simulink model "vegas13_fastnettest_250mhz_r1"  (Simulink 7.4)
settings: Solver=ode45  StartTime=0.0  StopTime=20000  RelTol=1e-3
undefined symbols (not defined in the file or in its folder): ROACH
libraries: xbsIndex_r4 x179, xps_library x20, casper_library_misc x18, dspsigops x16, casper_library_flow_control x4
(part 2 of 3)

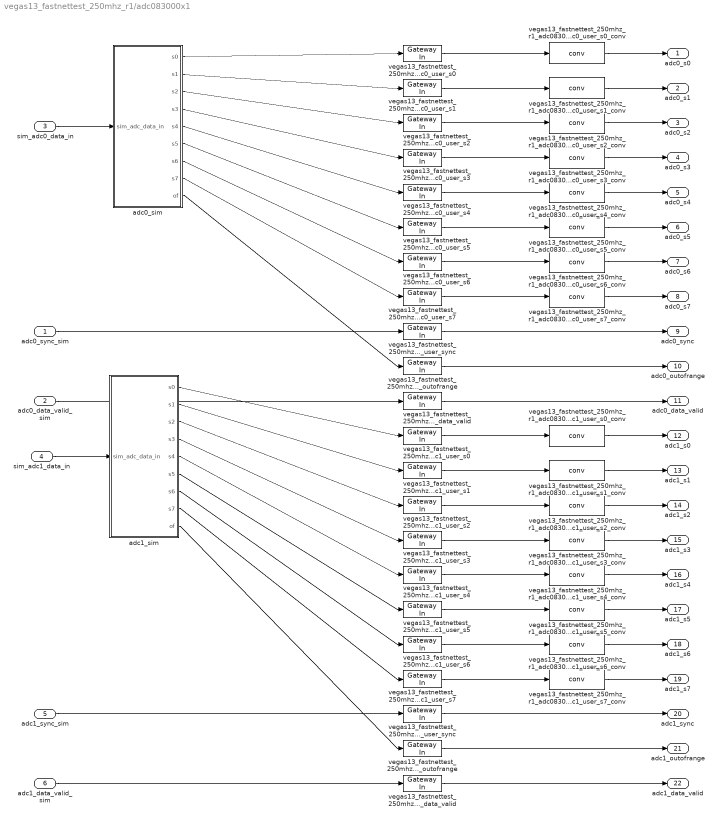
== system vegas13_fastnettest_250mhz_r1/adc083000x1 ==
  adc0_sync_sim : Inport  OutDataType=sfix(16)  OutScaling=2^0
  adc0_data_valid_sim : Inport  Port=2  OutDataType=sfix(16)  OutScaling=2^0
  sim_adc0_data_in : Inport  Port=3  OutDataType=fixdt(1, 16)  OutScaling=2^0
  sim_adc1_data_in : Inport  Port=4  OutDataType=fixdt(1, 16)  OutScaling=2^0
  adc1_sync_sim : Inport  Port=5  OutDataType=fixdt(1, 16)  OutScaling=2^0
  adc1_data_valid_sim : Inport  Port=6  OutDataType=fixdt(1, 16)  OutScaling=2^0
  adc0_sim : Subsystem  AncestorBlock=xps_library/ADCs/adc_sim  mask(adc_sim){nStreams=8, bit_width=8}
      mask prompts: nStreams "Number of Output Streams"; bit_width "Sample Bit Width"
      mask help:
      | This block simulates the behavior of a demuxed ADC, which takes
      | as input a waveform and returns digital samples in parallel at
      | a slower rate.
      |
      | This block is used to simulate the behavior
      mask init:
      | adc_sim_init(gcb, ...
      |     'nStreams', nStreams, ...
      |     'bit_width', bit_width);
  adc1_sim : Subsystem  AncestorBlock=xps_library/ADCs/adc_sim  mask(adc_sim){nStreams=8, bit_width=8}
      mask prompts: nStreams "Number of Output Streams"; bit_width "Sample Bit Width"
      mask help:
      | This block simulates the behavior of a demuxed ADC, which takes
      | as input a waveform and returns digital samples in parallel at
      | a slower rate.
      |
      | This block is used to simulate the behavior
      mask init:
      | adc_sim_init(gcb, ...
      |     'nStreams', nStreams, ...
      |     'bit_width', bit_width);
  vegas13_fastnettest_250mhz_r1_adc083000x1_adc0_user_data_valid : xbsIndex_r4/Gateway In  arith_type=Unsigned  n_bits=1  bin_pt=0  quantization="Round  (unbiased: +/- Inf)"  overflow=Saturate  period=1  dbl_ovrd=off  timing_constraint=None  locs_specified=off  LOCs={}  hdl_port=on  block_type=gatewayin
      settings: infoedit="Gateway in block.  Converts inputs of type Simulink integer, double and fixed point to  Xilinx fixed point type.<br><br>Hardware notes:  In hardware these blocks become top level input ports."  block_version=11.4
  vegas13_fastnettest_250mhz_r1_adc083000x1_adc0_user_outofrange : xbsIndex_r4/Gateway In  arith_type=Unsigned  n_bits=4  bin_pt=0  quantization="Round  (unbiased: +/- Inf)"  overflow=Saturate  period=1  dbl_ovrd=off  timing_constraint=None  locs_specified=off  LOCs={}  hdl_port=on  block_type=gatewayin
      settings: infoedit="Gateway in block.  Converts inputs of type Simulink integer, double and fixed point to  Xilinx fixed point type.<br><br>Hardware notes:  In hardware these blocks become top level input ports."  block_version=11.4
  vegas13_fastnettest_250mhz_r1_adc083000x1_adc0_user_s{0..7} (8 alike) : xbsIndex_r4/Gateway In  arith_type=Unsigned  n_bits=8  bin_pt=0  quantization="Round  (unbiased: +/- Inf)"  overflow=Saturate  period=1  dbl_ovrd=off  timing_constraint=None  locs_specified=off  LOCs={}  hdl_port=on  block_type=gatewayin
      settings: infoedit="Gateway in block.  Converts inputs of type Simulink integer, double and fixed point to  Xilinx fixed point type.<br><br>Hardware notes:  In hardware these blocks become top level input ports."  block_version=11.4
  vegas13_fastnettest_250mhz_r1_adc083000x1_adc0_user_s0_conv : xps_library/ADCs/conv  SystemSampleTime=-1  bit_width=8
  vegas13_fastnettest_250mhz_r1_adc083000x1_adc0_user_s1_conv : xps_library/ADCs/conv  SystemSampleTime=-1  bit_width=8
  vegas13_fastnettest_250mhz_r1_adc083000x1_adc0_user_s2_conv : xps_library/ADCs/conv  SystemSampleTime=-1  bit_width=8
  vegas13_fastnettest_250mhz_r1_adc083000x1_adc0_user_s3_conv : xps_library/ADCs/conv  SystemSampleTime=-1  bit_width=8
  vegas13_fastnettest_250mhz_r1_adc083000x1_adc0_user_s4_conv : xps_library/ADCs/conv  SystemSampleTime=-1  bit_width=8
  vegas13_fastnettest_250mhz_r1_adc083000x1_adc0_user_s5_conv : xps_library/ADCs/conv  SystemSampleTime=-1  bit_width=8
  vegas13_fastnettest_250mhz_r1_adc083000x1_adc0_user_s6_conv : xps_library/ADCs/conv  SystemSampleTime=-1  bit_width=8
  vegas13_fastnettest_250mhz_r1_adc083000x1_adc0_user_s7_conv : xps_library/ADCs/conv  SystemSampleTime=-1  bit_width=8
  vegas13_fastnettest_250mhz_r1_adc083000x1_adc0_user_sync : xbsIndex_r4/Gateway In  arith_type=Unsigned  n_bits=4  bin_pt=0  quantization="Round  (unbiased: +/- Inf)"  overflow=Saturate  period=1  dbl_ovrd=off  timing_constraint=None  locs_specified=off  LOCs={}  hdl_port=on  block_type=gatewayin
      settings: infoedit="Gateway in block.  Converts inputs of type Simulink integer, double and fixed point to  Xilinx fixed point type.<br><br>Hardware notes:  In hardware these blocks become top level input ports."  block_version=11.4
  vegas13_fastnettest_250mhz_r1_adc083000x1_adc1_user_data_valid : xbsIndex_r4/Gateway In  arith_type=Unsigned  n_bits=1  bin_pt=0  quantization="Round  (unbiased: +/- Inf)"  overflow=Saturate  period=1  dbl_ovrd=off  timing_constraint=None  locs_specified=off  LOCs={}  hdl_port=on  block_type=gatewayin
      settings: infoedit="Gateway in block.  Converts inputs of type Simulink integer, double and fixed point to  Xilinx fixed point type.<br><br>Hardware notes:  In hardware these blocks become top level input ports."  block_version=11.4
  vegas13_fastnettest_250mhz_r1_adc083000x1_adc1_user_outofrange : xbsIndex_r4/Gateway In  arith_type=Unsigned  n_bits=4  bin_pt=0  quantization="Round  (unbiased: +/- Inf)"  overflow=Saturate  period=1  dbl_ovrd=off  timing_constraint=None  locs_specified=off  LOCs={}  hdl_port=on  block_type=gatewayin
      settings: infoedit="Gateway in block.  Converts inputs of type Simulink integer, double and fixed point to  Xilinx fixed point type.<br><br>Hardware notes:  In hardware these blocks become top level input ports."  block_version=11.4
  vegas13_fastnettest_250mhz_r1_adc083000x1_adc1_user_s{0..7} (8 alike) : xbsIndex_r4/Gateway In  arith_type=Unsigned  n_bits=8  bin_pt=0  quantization="Round  (unbiased: +/- Inf)"  overflow=Saturate  period=1  dbl_ovrd=off  timing_constraint=None  locs_specified=off  LOCs={}  hdl_port=on  block_type=gatewayin
      settings: infoedit="Gateway in block.  Converts inputs of type Simulink integer, double and fixed point to  Xilinx fixed point type.<br><br>Hardware notes:  In hardware these blocks become top level input ports."  block_version=11.4
  vegas13_fastnettest_250mhz_r1_adc083000x1_adc1_user_s0_conv : xps_library/ADCs/conv  SystemSampleTime=-1  bit_width=8
  vegas13_fastnettest_250mhz_r1_adc083000x1_adc1_user_s1_conv : xps_library/ADCs/conv  SystemSampleTime=-1  bit_width=8
  vegas13_fastnettest_250mhz_r1_adc083000x1_adc1_user_s2_conv : xps_library/ADCs/conv  SystemSampleTime=-1  bit_width=8
  vegas13_fastnettest_250mhz_r1_adc083000x1_adc1_user_s3_conv : xps_library/ADCs/conv  SystemSampleTime=-1  bit_width=8
  vegas13_fastnettest_250mhz_r1_adc083000x1_adc1_user_s4_conv : xps_library/ADCs/conv  SystemSampleTime=-1  bit_width=8
  vegas13_fastnettest_250mhz_r1_adc083000x1_adc1_user_s5_conv : xps_library/ADCs/conv  SystemSampleTime=-1  bit_width=8
  vegas13_fastnettest_250mhz_r1_adc083000x1_adc1_user_s6_conv : xps_library/ADCs/conv  SystemSampleTime=-1  bit_width=8
  vegas13_fastnettest_250mhz_r1_adc083000x1_adc1_user_s7_conv : xps_library/ADCs/conv  SystemSampleTime=-1  bit_width=8
  vegas13_fastnettest_250mhz_r1_adc083000x1_adc1_user_sync : xbsIndex_r4/Gateway In  arith_type=Unsigned  n_bits=4  bin_pt=0  quantization="Round  (unbiased: +/- Inf)"  overflow=Saturate  period=1  dbl_ovrd=off  timing_constraint=None  locs_specified=off  LOCs={}  hdl_port=on  block_type=gatewayin
      settings: infoedit="Gateway in block.  Converts inputs of type Simulink integer, double and fixed point to  Xilinx fixed point type.<br><br>Hardware notes:  In hardware these blocks become top level input ports."  block_version=11.4
  adc0_s0 : Outport  OutDataType=fixdt(1, 16)  OutScaling=2^0
  adc0_s1 : Outport  Port=2  OutDataType=fixdt(1, 16)  OutScaling=2^0
  adc0_s2 : Outport  Port=3  OutDataType=fixdt(1, 16)  OutScaling=2^0
  adc0_s3 : Outport  Port=4  OutDataType=fixdt(1, 16)  OutScaling=2^0
  adc0_s4 : Outport  Port=5  OutDataType=fixdt(1, 16)  OutScaling=2^0
  adc0_s5 : Outport  Port=6  OutDataType=fixdt(1, 16)  OutScaling=2^0
  adc0_s6 : Outport  Port=7  OutDataType=fixdt(1, 16)  OutScaling=2^0
  adc0_s7 : Outport  Port=8  OutDataType=fixdt(1, 16)  OutScaling=2^0
  adc0_sync : Outport  Port=9  OutDataType=sfix(16)  OutScaling=2^0
  adc0_outofrange : Outport  Port=10  OutDataType=fixdt(1, 16)  OutScaling=2^0
  adc0_data_valid : Outport  Port=11  OutDataType=sfix(16)  OutScaling=2^0
  adc1_s0 : Outport  Port=12  OutDataType=fixdt(1, 16)  OutScaling=2^0
  adc1_s1 : Outport  Port=13  OutDataType=fixdt(1, 16)  OutScaling=2^0
  adc1_s2 : Outport  Port=14  OutDataType=fixdt(1, 16)  OutScaling=2^0
  adc1_s3 : Outport  Port=15  OutDataType=fixdt(1, 16)  OutScaling=2^0
  adc1_s4 : Outport  Port=16  OutDataType=fixdt(1, 16)  OutScaling=2^0
  adc1_s5 : Outport  Port=17  OutDataType=fixdt(1, 16)  OutScaling=2^0
  adc1_s6 : Outport  Port=18  OutDataType=fixdt(1, 16)  OutScaling=2^0
  adc1_s7 : Outport  Port=19  OutDataType=fixdt(1, 16)  OutScaling=2^0
  adc1_sync : Outport  Port=20  OutDataType=fixdt(1, 16)  OutScaling=2^0
  adc1_outofrange : Outport  Port=21  OutDataType=fixdt(1, 16)  OutScaling=2^0
  adc1_data_valid : Outport  Port=22  OutDataType=fixdt(1, 16)  OutScaling=2^0
  wires:
  sim_adc0_data_in/1 -> adc0_sim/1(sim_adc_data_in)
  sim_adc1_data_in/1 -> adc1_sim/1(sim_adc_data_in)
  adc0_sim/1(s0) -> vegas13_fastnettest_250mhz_r1_adc083000x1_adc0_user_s0/1
  vegas13_fastnettest_250mhz_r1_adc083000x1_adc0_user_s0/1 -> vegas13_fastnettest_250mhz_r1_adc083000x1_adc0_user_s0_conv/1
  vegas13_fastnettest_250mhz_r1_adc083000x1_adc0_user_s0_conv/1 -> adc0_s0/1
  adc0_sim/2(s1) -> vegas13_fastnettest_250mhz_r1_adc083000x1_adc0_user_s1/1
  vegas13_fastnettest_250mhz_r1_adc083000x1_adc0_user_s1/1 -> vegas13_fastnettest_250mhz_r1_adc083000x1_adc0_user_s1_conv/1
  vegas13_fastnettest_250mhz_r1_adc083000x1_adc0_user_s1_conv/1 -> adc0_s1/1
  adc0_sim/3(s2) -> vegas13_fastnettest_250mhz_r1_adc083000x1_adc0_user_s2/1
  vegas13_fastnettest_250mhz_r1_adc083000x1_adc0_user_s2/1 -> vegas13_fastnettest_250mhz_r1_adc083000x1_adc0_user_s2_conv/1
  vegas13_fastnettest_250mhz_r1_adc083000x1_adc0_user_s2_conv/1 -> adc0_s2/1
  adc0_sim/4(s3) -> vegas13_fastnettest_250mhz_r1_adc083000x1_adc0_user_s3/1
  vegas13_fastnettest_250mhz_r1_adc083000x1_adc0_user_s3/1 -> vegas13_fastnettest_250mhz_r1_adc083000x1_adc0_user_s3_conv/1
  vegas13_fastnettest_250mhz_r1_adc083000x1_adc0_user_s3_conv/1 -> adc0_s3/1
  adc0_sim/5(s4) -> vegas13_fastnettest_250mhz_r1_adc083000x1_adc0_user_s4/1
  vegas13_fastnettest_250mhz_r1_adc083000x1_adc0_user_s4/1 -> vegas13_fastnettest_250mhz_r1_adc083000x1_adc0_user_s4_conv/1
  vegas13_fastnettest_250mhz_r1_adc083000x1_adc0_user_s4_conv/1 -> adc0_s4/1
  adc0_sim/6(s5) -> vegas13_fastnettest_250mhz_r1_adc083000x1_adc0_user_s5/1
  vegas13_fastnettest_250mhz_r1_adc083000x1_adc0_user_s5/1 -> vegas13_fastnettest_250mhz_r1_adc083000x1_adc0_user_s5_conv/1
  vegas13_fastnettest_250mhz_r1_adc083000x1_adc0_user_s5_conv/1 -> adc0_s5/1
  adc0_sim/7(s6) -> vegas13_fastnettest_250mhz_r1_adc083000x1_adc0_user_s6/1
  vegas13_fastnettest_250mhz_r1_adc083000x1_adc0_user_s6/1 -> vegas13_fastnettest_250mhz_r1_adc083000x1_adc0_user_s6_conv/1
  vegas13_fastnettest_250mhz_r1_adc083000x1_adc0_user_s6_conv/1 -> adc0_s6/1
  adc0_sim/8(s7) -> vegas13_fastnettest_250mhz_r1_adc083000x1_adc0_user_s7/1
  vegas13_fastnettest_250mhz_r1_adc083000x1_adc0_user_s7/1 -> vegas13_fastnettest_250mhz_r1_adc083000x1_adc0_user_s7_conv/1
  vegas13_fastnettest_250mhz_r1_adc083000x1_adc0_user_s7_conv/1 -> adc0_s7/1
  adc0_sync_sim/1 -> vegas13_fastnettest_250mhz_r1_adc083000x1_adc0_user_sync/1
  vegas13_fastnettest_250mhz_r1_adc083000x1_adc0_user_sync/1 -> adc0_sync/1
  adc0_sim/9(of) -> vegas13_fastnettest_250mhz_r1_adc083000x1_adc0_user_outofrange/1
  vegas13_fastnettest_250mhz_r1_adc083000x1_adc0_user_outofrange/1 -> adc0_outofrange/1
  adc0_data_valid_sim/1 -> vegas13_fastnettest_250mhz_r1_adc083000x1_adc0_user_data_valid/1
  vegas13_fastnettest_250mhz_r1_adc083000x1_adc0_user_data_valid/1 -> adc0_data_valid/1
  adc1_sim/1(s0) -> vegas13_fastnettest_250mhz_r1_adc083000x1_adc1_user_s0/1
  vegas13_fastnettest_250mhz_r1_adc083000x1_adc1_user_s0/1 -> vegas13_fastnettest_250mhz_r1_adc083000x1_adc1_user_s0_conv/1
  vegas13_fastnettest_250mhz_r1_adc083000x1_adc1_user_s0_conv/1 -> adc1_s0/1
  adc1_sim/2(s1) -> vegas13_fastnettest_250mhz_r1_adc083000x1_adc1_user_s1/1
  vegas13_fastnettest_250mhz_r1_adc083000x1_adc1_user_s1/1 -> vegas13_fastnettest_250mhz_r1_adc083000x1_adc1_user_s1_conv/1
  vegas13_fastnettest_250mhz_r1_adc083000x1_adc1_user_s1_conv/1 -> adc1_s1/1
  adc1_sim/3(s2) -> vegas13_fastnettest_250mhz_r1_adc083000x1_adc1_user_s2/1
  vegas13_fastnettest_250mhz_r1_adc083000x1_adc1_user_s2/1 -> vegas13_fastnettest_250mhz_r1_adc083000x1_adc1_user_s2_conv/1
  vegas13_fastnettest_250mhz_r1_adc083000x1_adc1_user_s2_conv/1 -> adc1_s2/1
  adc1_sim/4(s3) -> vegas13_fastnettest_250mhz_r1_adc083000x1_adc1_user_s3/1
  vegas13_fastnettest_250mhz_r1_adc083000x1_adc1_user_s3/1 -> vegas13_fastnettest_250mhz_r1_adc083000x1_adc1_user_s3_conv/1
  vegas13_fastnettest_250mhz_r1_adc083000x1_adc1_user_s3_conv/1 -> adc1_s3/1
  adc1_sim/5(s4) -> vegas13_fastnettest_250mhz_r1_adc083000x1_adc1_user_s4/1
  vegas13_fastnettest_250mhz_r1_adc083000x1_adc1_user_s4/1 -> vegas13_fastnettest_250mhz_r1_adc083000x1_adc1_user_s4_conv/1
  vegas13_fastnettest_250mhz_r1_adc083000x1_adc1_user_s4_conv/1 -> adc1_s4/1
  adc1_sim/6(s5) -> vegas13_fastnettest_250mhz_r1_adc083000x1_adc1_user_s5/1
  vegas13_fastnettest_250mhz_r1_adc083000x1_adc1_user_s5/1 -> vegas13_fastnettest_250mhz_r1_adc083000x1_adc1_user_s5_conv/1
  vegas13_fastnettest_250mhz_r1_adc083000x1_adc1_user_s5_conv/1 -> adc1_s5/1
  adc1_sim/7(s6) -> vegas13_fastnettest_250mhz_r1_adc083000x1_adc1_user_s6/1
  vegas13_fastnettest_250mhz_r1_adc083000x1_adc1_user_s6/1 -> vegas13_fastnettest_250mhz_r1_adc083000x1_adc1_user_s6_conv/1
  vegas13_fastnettest_250mhz_r1_adc083000x1_adc1_user_s6_conv/1 -> adc1_s6/1
  adc1_sim/8(s7) -> vegas13_fastnettest_250mhz_r1_adc083000x1_adc1_user_s7/1
  vegas13_fastnettest_250mhz_r1_adc083000x1_adc1_user_s7/1 -> vegas13_fastnettest_250mhz_r1_adc083000x1_adc1_user_s7_conv/1
  vegas13_fastnettest_250mhz_r1_adc083000x1_adc1_user_s7_conv/1 -> adc1_s7/1
  adc1_sync_sim/1 -> vegas13_fastnettest_250mhz_r1_adc083000x1_adc1_user_sync/1
  vegas13_fastnettest_250mhz_r1_adc083000x1_adc1_user_sync/1 -> adc1_sync/1
  adc1_sim/9(of) -> vegas13_fastnettest_250mhz_r1_adc083000x1_adc1_user_outofrange/1
  vegas13_fastnettest_250mhz_r1_adc083000x1_adc1_user_outofrange/1 -> adc1_outofrange/1
  adc1_data_valid_sim/1 -> vegas13_fastnettest_250mhz_r1_adc083000x1_adc1_user_data_valid/1
  vegas13_fastnettest_250mhz_r1_adc083000x1_adc1_user_data_valid/1 -> adc1_data_valid/1

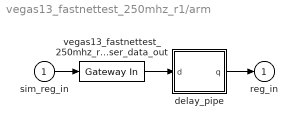
== system vegas13_fastnettest_250mhz_r1/arm ==
  sim_reg_in : Inport
  delay_pipe : Subsystem
  vegas13_fastnettest_250mhz_r1_arm_user_data_out : xbsIndex_r4/Gateway In  arith_type=Unsigned  n_bits=32  bin_pt=0  quantization="Round  (unbiased: +/- Inf)"  overflow=Saturate  period=1  dbl_ovrd=off  timing_constraint=None  locs_specified=off  LOCs={}  hdl_port=on  block_type=gatewayin
      settings: infoedit="Gateway in block.  Converts inputs of type Simulink integer, double and fixed point to  Xilinx fixed point type.<br><br>Hardware notes:  In hardware these blocks become top level input ports."  block_version=11.4
  reg_in : Outport
  wires:
  delay_pipe/1(q) -> reg_in/1
  vegas13_fastnettest_250mhz_r1_arm_user_data_out/1 -> delay_pipe/1(d)
  sim_reg_in/1 -> vegas13_fastnettest_250mhz_r1_arm_user_data_out/1

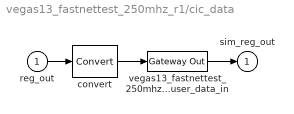
== system vegas13_fastnettest_250mhz_r1/cic_data ==
  reg_out : Inport
  convert : xbsIndex_r4/Convert  arith_type=Unsigned  n_bits=32  bin_pt=0  quantization=Truncate  overflow=Wrap  latency=0  dbl_ovrd=off  pipeline=off  block_type=convert
      settings: block_version=11.4
  vegas13_fastnettest_250mhz_r1_cic_data_user_data_in : xbsIndex_r4/Gateway Out  hdl_port=on  timing_constraint=None  locs_specified=off  LOCs={}  block_type=gatewayout
      settings: infoedit="Gateway out block.  Converts Xilinx fixed point inputs into ouputs of type Simulink integer, double, or fixed point.<br><br>Hardware notes:  In hardware these blocks become top level output ports or are discarded, depending on how they are configured."  block_version=11.4
  sim_reg_out : Outport
  wires:
  vegas13_fastnettest_250mhz_r1_cic_data_user_data_in/1 -> sim_reg_out/1
  convert/1 -> vegas13_fastnettest_250mhz_r1_cic_data_user_data_in/1
  reg_out/1 -> convert/1

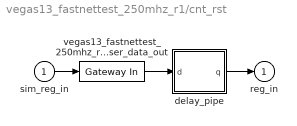
== system vegas13_fastnettest_250mhz_r1/cnt_rst ==
  sim_reg_in : Inport
  delay_pipe : Subsystem
  vegas13_fastnettest_250mhz_r1_cnt_rst_user_data_out : xbsIndex_r4/Gateway In  arith_type=Unsigned  n_bits=32  bin_pt=0  quantization="Round  (unbiased: +/- Inf)"  overflow=Saturate  period=1  dbl_ovrd=off  timing_constraint=None  locs_specified=off  LOCs={}  hdl_port=on  block_type=gatewayin
      settings: infoedit="Gateway in block.  Converts inputs of type Simulink integer, double and fixed point to  Xilinx fixed point type.<br><br>Hardware notes:  In hardware these blocks become top level input ports."  block_version=11.4
  reg_in : Outport
  wires:
  delay_pipe/1(q) -> reg_in/1
  vegas13_fastnettest_250mhz_r1_cnt_rst_user_data_out/1 -> delay_pipe/1(d)
  sim_reg_in/1 -> vegas13_fastnettest_250mhz_r1_cnt_rst_user_data_out/1

== system vegas13_fastnettest_250mhz_r1/dest_ip ==
  sim_reg_in : Inport
  delay_pipe : Subsystem
  vegas13_fastnettest_250mhz_r1_dest_ip_user_data_out : xbsIndex_r4/Gateway In  arith_type=Unsigned  n_bits=32  bin_pt=0  quantization="Round  (unbiased: +/- Inf)"  overflow=Saturate  period=1  dbl_ovrd=off  timing_constraint=None  locs_specified=off  LOCs={}  hdl_port=on  block_type=gatewayin
      settings: infoedit="Gateway in block.  Converts inputs of type Simulink integer, double and fixed point to  Xilinx fixed point type.<br><br>Hardware notes:  In hardware these blocks become top level input ports."  block_version=11.4
  reg_in : Outport
  wires:
  delay_pipe/1(q) -> reg_in/1
  vegas13_fastnettest_250mhz_r1_dest_ip_user_data_out/1 -> delay_pipe/1(d)
  sim_reg_in/1 -> vegas13_fastnettest_250mhz_r1_dest_ip_user_data_out/1

== system vegas13_fastnettest_250mhz_r1/dest_port ==
  sim_reg_in : Inport
  delay_pipe : Subsystem
  vegas13_fastnettest_250mhz_r1_dest_port_user_data_out : xbsIndex_r4/Gateway In  arith_type=Unsigned  n_bits=32  bin_pt=0  quantization="Round  (unbiased: +/- Inf)"  overflow=Saturate  period=1  dbl_ovrd=off  timing_constraint=None  locs_specified=off  LOCs={}  hdl_port=on  block_type=gatewayin
      settings: infoedit="Gateway in block.  Converts inputs of type Simulink integer, double and fixed point to  Xilinx fixed point type.<br><br>Hardware notes:  In hardware these blocks become top level input ports."  block_version=11.4
  reg_in : Outport
  wires:
  delay_pipe/1(q) -> reg_in/1
  vegas13_fastnettest_250mhz_r1_dest_port_user_data_out/1 -> delay_pipe/1(d)
  sim_reg_in/1 -> vegas13_fastnettest_250mhz_r1_dest_port_user_data_out/1

== system vegas13_fastnettest_250mhz_r1/eth_rst ==
  sim_reg_in : Inport
  delay_pipe : Subsystem
  vegas13_fastnettest_250mhz_r1_eth_rst_user_data_out : xbsIndex_r4/Gateway In  arith_type=Unsigned  n_bits=32  bin_pt=0  quantization="Round  (unbiased: +/- Inf)"  overflow=Saturate  period=1  dbl_ovrd=off  timing_constraint=None  locs_specified=off  LOCs={}  hdl_port=on  block_type=gatewayin
      settings: infoedit="Gateway in block.  Converts inputs of type Simulink integer, double and fixed point to  Xilinx fixed point type.<br><br>Hardware notes:  In hardware these blocks become top level input ports."  block_version=11.4
  reg_in : Outport
  wires:
  delay_pipe/1(q) -> reg_in/1
  vegas13_fastnettest_250mhz_r1_eth_rst_user_data_out/1 -> delay_pipe/1(d)
  sim_reg_in/1 -> vegas13_fastnettest_250mhz_r1_eth_rst_user_data_out/1

== system vegas13_fastnettest_250mhz_r1/ext_sync_ctr ==
  reg_out : Inport
  convert : xbsIndex_r4/Convert  arith_type=Unsigned  n_bits=32  bin_pt=0  quantization=Truncate  overflow=Wrap  latency=0  dbl_ovrd=off  pipeline=off  block_type=convert
      settings: block_version=11.4
  vegas13_fastnettest_250mhz_r1_ext_sync_ctr_user_data_in : xbsIndex_r4/Gateway Out  hdl_port=on  timing_constraint=None  locs_specified=off  LOCs={}  block_type=gatewayout
      settings: infoedit="Gateway out block.  Converts Xilinx fixed point inputs into ouputs of type Simulink integer, double, or fixed point.<br><br>Hardware notes:  In hardware these blocks become top level output ports or are discarded, depending on how they are configured."  block_version=11.4
  sim_reg_out : Outport
  wires:
  vegas13_fastnettest_250mhz_r1_ext_sync_ctr_user_data_in/1 -> sim_reg_out/1
  convert/1 -> vegas13_fastnettest_250mhz_r1_ext_sync_ctr_user_data_in/1
  reg_out/1 -> convert/1

== system vegas13_fastnettest_250mhz_r1/ip_select ==
  sim_reg_in : Inport
  delay_pipe : Subsystem
  vegas13_fastnettest_250mhz_r1_ip_select_user_data_out : xbsIndex_r4/Gateway In  arith_type=Unsigned  n_bits=32  bin_pt=0  quantization="Round  (unbiased: +/- Inf)"  overflow=Saturate  period=1  dbl_ovrd=off  timing_constraint=None  locs_specified=off  LOCs={}  hdl_port=on  block_type=gatewayin
      settings: infoedit="Gateway in block.  Converts inputs of type Simulink integer, double and fixed point to  Xilinx fixed point type.<br><br>Hardware notes:  In hardware these blocks become top level input ports."  block_version=11.4
  reg_in : Outport
  wires:
  delay_pipe/1(q) -> reg_in/1
  vegas13_fastnettest_250mhz_r1_ip_select_user_data_out/1 -> delay_pipe/1(d)
  sim_reg_in/1 -> vegas13_fastnettest_250mhz_r1_ip_select_user_data_out/1

== system vegas13_fastnettest_250mhz_r1/pkt_data ==
  reg_out : Inport
  convert : xbsIndex_r4/Convert  arith_type=Unsigned  n_bits=32  bin_pt=0  quantization=Truncate  overflow=Wrap  latency=0  dbl_ovrd=off  pipeline=off  block_type=convert
      settings: block_version=11.4
  vegas13_fastnettest_250mhz_r1_pkt_data_user_data_in : xbsIndex_r4/Gateway Out  hdl_port=on  timing_constraint=None  locs_specified=off  LOCs={}  block_type=gatewayout
      settings: infoedit="Gateway out block.  Converts Xilinx fixed point inputs into ouputs of type Simulink integer, double, or fixed point.<br><br>Hardware notes:  In hardware these blocks become top level output ports or are discarded, depending on how they are configured."  block_version=11.4
  sim_reg_out : Outport
  wires:
  vegas13_fastnettest_250mhz_r1_pkt_data_user_data_in/1 -> sim_reg_out/1
  convert/1 -> vegas13_fastnettest_250mhz_r1_pkt_data_user_data_in/1
  reg_out/1 -> convert/1

== system vegas13_fastnettest_250mhz_r1/port_select ==
  sim_reg_in : Inport
  delay_pipe : Subsystem
  vegas13_fastnettest_250mhz_r1_port_select_user_data_out : xbsIndex_r4/Gateway In  arith_type=Unsigned  n_bits=32  bin_pt=0  quantization="Round  (unbiased: +/- Inf)"  overflow=Saturate  period=1  dbl_ovrd=off  timing_constraint=None  locs_specified=off  LOCs={}  hdl_port=on  block_type=gatewayin
      settings: infoedit="Gateway in block.  Converts inputs of type Simulink integer, double and fixed point to  Xilinx fixed point type.<br><br>Hardware notes:  In hardware these blocks become top level input ports."  block_version=11.4
  reg_in : Outport
  wires:
  delay_pipe/1(q) -> reg_in/1
  vegas13_fastnettest_250mhz_r1_port_select_user_data_out/1 -> delay_pipe/1(d)
  sim_reg_in/1 -> vegas13_fastnettest_250mhz_r1_port_select_user_data_out/1

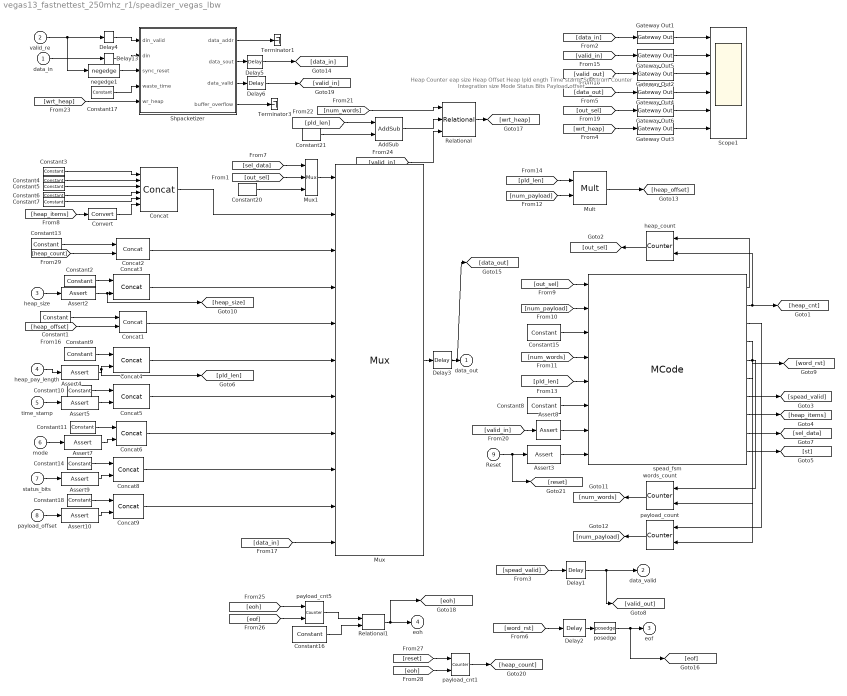
== system vegas13_fastnettest_250mhz_r1/speadizer_vegas_lbw ==
  note: Heap Counter
      | eap size
      | Heap Offset
      | Heap lpld ength
      | Time stamp
      | Spectrum Counter
      | Integration size
      | Mode
      | Status Bits
      | Payload offset
  data_in : Inport
  valid_re : Inport  Port=2
  heap_size : Inport  Port=3
  heap_pay_length : Inport  Port=4
  time_stamp : Inport  Port=5
  mode : Inport  Port=6
  status_bits : Inport  Port=7
  payload_offset : Inport  Port=8
  Reset : Inport  Port=9
  AddSub : xbsIndex_r4/AddSub  mode=Subtraction  use_carryin=off  use_carryout=off  en=off  latency=0  precision=Full  arith_type=Unsigned  n_bits=16  bin_pt=14  quantization=Truncate  overflow=Wrap  dbl_ovrd=off  use_behavioral_HDL=off  hw_selection=Fabric  pipelined=off  block_type=addsub
  Assert{2,4..5,7,9..10} (6 alike) : xbsIndex_r4/Assert  assert_type=on  type_source=Explicitly  arith_type=Unsigned  n_bits=spead_lsw  bin_pt=0  assert_rate=off  rate_source=Explicitly  period=1  output_port=on  block_type=assert
      settings: block_version=11.4
  Assert3 : xbsIndex_r4/Assert  assert_type=on  type_source=Explicitly  arith_type=Boolean  n_bits=spead_lsw  bin_pt=0  assert_rate=on  rate_source=Explicitly  period=1  output_port=on  block_type=assert
      settings: block_version=11.4
  Assert8 : xbsIndex_r4/Assert  assert_type=on  type_source=Explicitly  arith_type=Boolean  n_bits=spead_lsw  bin_pt=0  assert_rate=on  rate_source=Explicitly  period=1  output_port=on  block_type=assert
      settings: block_version=11.4
  Concat : xbsIndex_r4/Concat  num_inputs=6  dbl_ovrd=off  block_type=concat
  Concat{1..6,8..9} (8 alike) : xbsIndex_r4/Concat  num_inputs=2  dbl_ovrd=off  block_type=concat
  Constant1 : xbsIndex_r4/Constant  arith_type=Unsigned  const=8388608+3  n_bits=spead_msw  bin_pt=0  explicit_period=on  period=1  equ=P=C  opselect=C  inp2=PCIN>>17  opr=+  inp1=P  carry=CIN  dbl_ovrd=off  block_type=constant
      settings: block_version=11.4
  Constant10 : xbsIndex_r4/Constant  arith_type=Unsigned  const=8388608+32  n_bits=spead_msw  bin_pt=0  explicit_period=on  period=1  equ=P=C  opselect=C  inp2=PCIN>>17  opr=+  inp1=P  carry=CIN  dbl_ovrd=off  block_type=constant
      settings: block_version=11.4
  Constant11 : xbsIndex_r4/Constant  arith_type=Unsigned  const=8388608+33  n_bits=spead_msw  bin_pt=0  explicit_period=on  period=1  equ=P=C  opselect=C  inp2=PCIN>>17  opr=+  inp1=P  carry=CIN  dbl_ovrd=off  block_type=constant
      settings: block_version=11.4
  Constant13 : xbsIndex_r4/Constant  arith_type=Unsigned  const=8388608+1  n_bits=spead_msw  bin_pt=0  explicit_period=on  period=1  equ=P=C  opselect=C  inp2=PCIN>>17  opr=+  inp1=P  carry=CIN  dbl_ovrd=off  block_type=constant
      settings: block_version=11.4
  Constant14 : xbsIndex_r4/Constant  arith_type=Unsigned  const=8388608+34  n_bits=spead_msw  bin_pt=0  explicit_period=on  period=1  equ=P=C  opselect=C  inp2=PCIN>>17  opr=+  inp1=P  carry=CIN  dbl_ovrd=off  block_type=constant
      settings: block_version=11.4
  Constant15 : xbsIndex_r4/Constant  arith_type=Unsigned  const=num_items+5  n_bits=8  bin_pt=0  explicit_period=on  period=1  equ=P=C  opselect=C  inp2=PCIN>>17  opr=+  inp1=P  carry=CIN  dbl_ovrd=off  block_type=constant
      settings: block_version=11.4
  Constant16 : xbsIndex_r4/Constant  arith_type=Unsigned  const=num_payloads  n_bits=4  bin_pt=0  explicit_period=on  period=1  equ=P=C  opselect=C  inp2=PCIN>>17  opr=+  inp1=P  carry=CIN  dbl_ovrd=off  block_type=constant
      settings: block_version=11.4
  Constant17 : xbsIndex_r4/Constant  arith_type=Unsigned  const=pktzr_waste_time  n_bits=7  bin_pt=0  explicit_period=on  period=1  equ=P=C  opselect=C  inp2=PCIN>>17  opr=+  inp1=P  carry=CIN  dbl_ovrd=off  block_type=constant
  Constant18 : xbsIndex_r4/Constant  arith_type=Unsigned  const=0+35  n_bits=spead_msw  bin_pt=0  explicit_period=on  period=1  equ=P=C  opselect=C  inp2=PCIN>>17  opr=+  inp1=P  carry=CIN  dbl_ovrd=off  block_type=constant
      settings: block_version=11.4
  Constant2 : xbsIndex_r4/Constant  arith_type=Unsigned  const=8388608+2  n_bits=spead_msw  bin_pt=0  explicit_period=on  period=1  equ=P=C  opselect=C  inp2=PCIN>>17  opr=+  inp1=P  carry=CIN  dbl_ovrd=off  block_type=constant
      settings: block_version=11.4
  Constant20 : xbsIndex_r4/Constant  arith_type=Unsigned  const=num_items+5  n_bits=4  bin_pt=0  explicit_period=on  period=1  equ=P=C  opselect=C  inp2=PCIN>>17  opr=+  inp1=P  carry=CIN  dbl_ovrd=off  block_type=constant
      settings: block_version=11.4
  Constant21 : xbsIndex_r4/Constant  arith_type=Unsigned  const=16  n_bits=5  bin_pt=0  explicit_period=on  period=1  equ=P=C  opselect=C  inp2=PCIN>>17  opr=+  inp1=P  carry=CIN  dbl_ovrd=off  block_type=constant
      settings: block_version=11.4
  Constant3 : xbsIndex_r4/Constant  arith_type=Unsigned  const=83  n_bits=8  bin_pt=0  explicit_period=on  period=1  equ=P=C  opselect=C  inp2=PCIN>>17  opr=+  inp1=P  carry=CIN  dbl_ovrd=off  block_type=constant
      settings: block_version=11.4
  Constant4 : xbsIndex_r4/Constant  arith_type=Unsigned  const=4  n_bits=8  bin_pt=0  explicit_period=on  period=1  equ=P=C  opselect=C  inp2=PCIN>>17  opr=+  inp1=P  carry=CIN  dbl_ovrd=off  block_type=constant
      settings: block_version=11.4
  Constant5 : xbsIndex_r4/Constant  arith_type=Unsigned  const=3  n_bits=8  bin_pt=0  explicit_period=on  period=1  equ=P=C  opselect=C  inp2=PCIN>>17  opr=+  inp1=P  carry=CIN  dbl_ovrd=off  block_type=constant
      settings: block_version=11.4
  Constant6 : xbsIndex_r4/Constant  arith_type=Unsigned  const=5  n_bits=8  bin_pt=0  explicit_period=on  period=1  equ=P=C  opselect=C  inp2=PCIN>>17  opr=+  inp1=P  carry=CIN  dbl_ovrd=off  block_type=constant
      settings: block_version=11.4
  Constant7 : xbsIndex_r4/Constant  arith_type=Unsigned  const=0  n_bits=16  bin_pt=0  explicit_period=on  period=1  equ=P=C  opselect=C  inp2=PCIN>>17  opr=+  inp1=P  carry=CIN  dbl_ovrd=off  block_type=constant
      settings: block_version=11.4
  Constant8 : xbsIndex_r4/Constant  arith_type=Unsigned  const=num_payloads  n_bits=8  bin_pt=0  explicit_period=on  period=1  equ=P=C  opselect=C  inp2=PCIN>>17  opr=+  inp1=P  carry=CIN  dbl_ovrd=off  block_type=constant
      settings: block_version=11.4
  Constant9 : xbsIndex_r4/Constant  arith_type=Unsigned  const=8388608+4  n_bits=spead_msw  bin_pt=0  explicit_period=on  period=1  equ=P=C  opselect=C  inp2=PCIN>>17  opr=+  inp1=P  carry=CIN  dbl_ovrd=off  block_type=constant
      settings: block_version=11.4
  Convert : xbsIndex_r4/Convert  arith_type=Unsigned  n_bits=16  bin_pt=0  quantization=Truncate  overflow=Wrap  latency=0  dbl_ovrd=off  pipeline=off  block_type=convert
      settings: block_version=11.4
  Delay1 : xbsIndex_r4/Delay  en=off  latency=2  dbl_ovrd=off  reg_retiming=on  block_type=delay
      settings: block_version=11.4
  Delay13 : xbsIndex_r4/Delay  en=off  latency=2  dbl_ovrd=off  reg_retiming=off  block_type=delay
      settings: block_version=11.4
  Delay2 : xbsIndex_r4/Delay  en=off  latency=1  dbl_ovrd=off  reg_retiming=on  block_type=delay
      settings: block_version=11.4
  Delay3 : xbsIndex_r4/Delay  en=off  latency=1  dbl_ovrd=off  reg_retiming=on  block_type=delay
      settings: block_version=11.4
  Delay4 : xbsIndex_r4/Delay  en=off  latency=2  dbl_ovrd=off  reg_retiming=off  block_type=delay
      settings: block_version=11.4
  Delay5 : xbsIndex_r4/Delay  en=off  latency=3  dbl_ovrd=off  reg_retiming=on  block_type=delay
      settings: block_version=11.4
  Delay6 : xbsIndex_r4/Delay  en=off  latency=3  dbl_ovrd=off  reg_retiming=on  block_type=delay
      settings: block_version=11.4
  Gateway Out{1..6} (6 alike) : xbsIndex_r4/Gateway Out  hdl_port=on  timing_constraint=None  locs_specified=off  LOCs={}  block_type=gatewayout
      settings: infoedit="Gateway out block.  Converts Xilinx fixed point inputs into ouputs of type Simulink integer, double, or fixed point.<br><br>Hardware notes:  In hardware these blocks become top level output ports or are discarded, depending on how they are configured."  block_version=11.4
  Mult : xbsIndex_r4/Mult  precision=User Defined  arith_type=Unsigned  n_bits=40  bin_pt=0  quantization=Truncate  overflow=Wrap  en=off  latency=6  dbl_ovrd=off  use_behavioral_HDL=off  opt=Speed  use_embedded=on  optimum_pipeline=off  pipeline=on  use_rpm=on  placement_style=Triangular  block_type=mult
      settings: block_version=11.4
  Mux : xbsIndex_r4/Mux  inputs=10  en=off  latency=1  precision=User Defined  arith_type=Unsigned  n_bits=64  bin_pt=0  quantization=Truncate  overflow=Wrap  dbl_ovrd=off  block_type=mux
      settings: block_version=11.4
  Mux1 : xbsIndex_r4/Mux  inputs=2  en=off  latency=0  precision=Full  arith_type="Signed  (2's comp)"  n_bits=8  bin_pt=2  quantization=Truncate  overflow=Wrap  dbl_ovrd=off  block_type=mux
      settings: block_version=11.4
  Relational : xbsIndex_r4/Relational  mode=a>=b  en=on  latency=1  dbl_ovrd=off  block_type=relational
  Relational1 : xbsIndex_r4/Relational  mode=a=b  en=off  latency=0  dbl_ovrd=off  block_type=relational
  Scope1 : Scope  NumInputPorts=6
      settings: TimeRange=1000  YMin=0~0~0~0~0~0  YMax=40~1~1~1e+19~1~20  SaveName=ScopeData2  MaxDataPoints=10000
  Shpacketizer : Subsystem  AncestorBlock=gbt_library/Spacketizer  mask(shpacketizer){pin_width=256, sout_width=64, fifo_depth=128, total_words=1024}
      mask prompts: pin_width "Parallel Input Width"; sout_width "Serial Output Width"; fifo_depth "FIFO depth"; total_words "Total number of data points"
      mask help:
      | This block is intended to serialize data that is 'bursty', that is,
      | the average data rate is small but per cycle the data is highly
      | parallel and can contain many points simultaneously.  This situation
      | is common with the streaming CASPER FFTs and related blocks.
      |
      | The serialization buffers the data when valid and independently
      | serializes the data when the buffer is non-empty.  For convenience, the
      | data is counted as it is serialized and signals exist to indicate
      | that the serial output is valid or that a buffer overflow has occured.  The
      | block will not stop in the case of an overflow, and the overflow
      | signal is not held high after it occurs.
      |
      | For example usage, see 'roach_spec_2adc_borph' in 'SVNROOT/trunk/projects/roach_spec/'
      | or the test case in 'SVNROOT/trunk/mlib_devel_10_1/Tests/packetizer_test.mdl'
      |
      | For extended documentation, please see the CASPER wiki
      mask init:
      | shpacketizer_init(gcb, 'pin_width', pin_width, 'sout_width', sout_width, 'total_words', total_words, 'fifo_depth', fifo_depth)
      | % packetizer_init(gcb, ...
      | %     'pin_width', pin_width, ...
      | %     'sout_width', sout_width, ...
      | %   %  'fifo_depth', fifo_depth, ...
      | %     'total_words', total_words);
      settings: AttributesFormatString=|
      | Parallel Input Width: 256
      | Serial Output Width: 64
      mask StyleString: edit,edit,popup(16|32|64|128|256|512|1K|2K|4K|8K|16K|32K|64K),edit
  Terminator1 : Terminator
  Terminator3 : Terminator
  heap_count : xbsIndex_r4/Counter  cnt_type=Free Running  cnt_to=Inf  operation=Up  start_count=0  cnt_by_val=1  arith_type=Unsigned  n_bits=4  bin_pt=0  load_pin=off  rst=on  en=on  explicit_period=on  period=1  dbl_ovrd=off  use_behavioral_HDL=off  implementation=Fabric  block_type=counter
      settings: block_version=11.4
  negedge1 : casper_library_misc/negedge  Tag=Rising Edge Detector  SystemSampleTime=-1
  payload_cnt1 : xbsIndex_r4/Counter  cnt_type=Free Running  cnt_to=0  operation=Up  start_count=1024  cnt_by_val=1  arith_type=Unsigned  n_bits=40  bin_pt=0  load_pin=off  rst=on  en=on  explicit_period=on  period=1  dbl_ovrd=off  use_behavioral_HDL=off  implementation=Fabric  use_rpm=on  block_type=counter
      settings: xl_area=[0, 0, 0, 0, 0, 0, 0]
  payload_cnt5 : xbsIndex_r4/Counter  cnt_type=Free Running  cnt_to=0  operation=Up  start_count=0  cnt_by_val=1  arith_type=Unsigned  n_bits=4  bin_pt=0  load_pin=off  rst=on  en=on  explicit_period=on  period=1  dbl_ovrd=off  use_behavioral_HDL=off  implementation=Fabric  use_rpm=on  block_type=counter
      settings: xl_area=[0, 0, 0, 0, 0, 0, 0]
  payload_count : xbsIndex_r4/Counter  cnt_type=Free Running  cnt_to=Inf  operation=Up  start_count=0  cnt_by_val=1  arith_type=Unsigned  n_bits=8  bin_pt=0  load_pin=off  rst=on  en=on  explicit_period=on  period=1  dbl_ovrd=off  use_behavioral_HDL=off  implementation=Fabric  block_type=counter
      settings: block_version=11.4
  posedge : casper_library_misc/posedge  Tag=Rising Edge Detector  SystemSampleTime=-1
  spead_fsm : xbsIndex_r4/MCode  mfname=spead_fsm  explicit_period=on  period=1  inputsTable={'boundInpExpr'=>['','','','5','','','','',''],'inputs'=>['head_count','num_payload_sent','total_header_len','min_header_len','num_words_sent','payload_len','total_num_payloads','data_valid_in','rst']}  outputsTable={'outputs'=>['head_count_rst','head_count_en','num_payload_rst','num_payload_en','words_sent_rst','words_sent_en','tge_valid','heap_elements','select_data','st'],'suppressOut'=>['off','off','off','off','off','off','off','off','off','off']}  dbl_ovrd=off  enable_stdout=off  enable_debug=off  suppress_output=on  defparams={'min_header_len',5}  hide_port_list={}  block_type=mcode
      settings: block_version=11.4
  words_count : xbsIndex_r4/Counter  cnt_type=Free Running  cnt_to=Inf  operation=Up  start_count=0  cnt_by_val=8  arith_type=Unsigned  n_bits=15  bin_pt=0  load_pin=off  rst=on  en=on  explicit_period=on  period=1  dbl_ovrd=off  use_behavioral_HDL=off  implementation=Fabric  block_type=counter
      settings: block_version=11.4
  data_out : Outport
  data_valid : Outport  Port=2
  eof : Outport  Port=3
  eoh : Outport  Port=4
  wires:
  [data_in] -> Mux/11
  payload_offset/1 -> Assert10/1
  status_bits/1 -> Assert9/1
  mode/1 -> Assert7/1
  Concat2/1 -> Mux/3
  [heap_count] -> Concat2/2
  Constant13/1 -> Concat2/1
  [eoh] -> payload_cnt1/2
  [reset] -> payload_cnt1/1
  payload_cnt1/1 -> [heap_count]
  payload_cnt5/1 -> Relational1/1
  Constant16/1 -> Relational1/2
  Relational1/1 -> [eoh], eoh/1
  [eof] -> payload_cnt5/2
  [eoh] -> payload_cnt5/1
  [valid_in] -> Relational/3
  Relational/1 -> [wrt_heap]
  AddSub/1 -> Relational/2
  Constant21/1 -> AddSub/2
  [pld_len] -> AddSub/1
  [num_words] -> Relational/1
  [wrt_heap] -> Shpacketizer/5(wr_heap)
  Delay13/1 -> Shpacketizer/2(din)
  negedge1/1 -> Shpacketizer/3(sync_reset)
  Constant17/1 -> Shpacketizer/4(waste_time)
  Delay4/1 -> Shpacketizer/1(din_valid)
  valid_re/1 -> negedge1/1, Delay4/1
  [valid_in] -> Assert8/1
  Delay6/1 -> [valid_in]
  Shpacketizer/3(data_valid) -> Delay6/1
  Delay5/1 -> [data_in]
  Shpacketizer/1(data_addr) -> Terminator1/1
  Shpacketizer/4(buffer_overflow) -> Terminator3/1
  data_in/1 -> Delay13/1
  Shpacketizer/2(data_sout) -> Delay5/1
  [wrt_heap] -> Gateway Out3/1
  [sel_data] -> Mux1/1
  [out_sel] -> Mux1/2
  Mux/1 -> Delay3/1
  Delay3/1 -> [data_out], data_out/1
  Mult/1 -> [heap_offset]
  [pld_len] -> Mult/1
  [num_payload] -> Mult/2
  Delay2/1 -> posedge/1
  Constant15/1 -> spead_fsm/3
  [num_words] -> spead_fsm/4
  [pld_len] -> spead_fsm/5
  Constant8/1 -> spead_fsm/6
  Assert8/1 -> spead_fsm/7
  Assert3/1 -> spead_fsm/8
  [word_rst] -> Delay2/1
  posedge/1 -> [eof], eof/1
  Gateway Out5/1 -> Scope1/2
  [valid_in] -> Gateway Out5/1
  [num_payload] -> spead_fsm/2
  [out_sel] -> spead_fsm/1
  heap_count/1 -> [out_sel]
  payload_count/1 -> [num_payload]
  words_count/1 -> [num_words]
  Convert/1 -> Concat/6
  [heap_items] -> Convert/1
  spead_fsm/9 -> [sel_data]
  spead_fsm/10 -> [st]
  Mux1/1 -> Mux/1
  Constant20/1 -> Mux1/3
  [data_out] -> Gateway Out4/1
  Gateway Out4/1 -> Scope1/4
  Gateway Out3/1 -> Scope1/6
  Gateway Out1/1 -> Scope1/1
  [data_in] -> Gateway Out1/1
  Reset/1 -> [reset], Assert3/1
  [heap_offset] -> Concat1/2
  spead_fsm/8 -> [heap_items]
  spead_fsm/7 -> [spead_valid]
  spead_fsm/2 -> [heap_cnt], heap_count/2
  spead_fsm/1 -> heap_count/1
  spead_fsm/4 -> [word_rst], payload_count/2
  spead_fsm/3 -> payload_count/1
  spead_fsm/6 -> words_count/2
  spead_fsm/5 -> words_count/1
  Gateway Out6/1 -> Scope1/5
  Gateway Out2/1 -> Scope1/3
  Concat8/1 -> Mux/9
  Constant14/1 -> Concat8/1
  Assert9/1 -> Concat8/2
  Concat5/1 -> Mux/7
  Concat6/1 -> Mux/8
  Constant11/1 -> Concat6/1
  Assert7/1 -> Concat6/2
  Concat9/1 -> Mux/10
  Concat1/1 -> Mux/5
  Constant1/1 -> Concat1/1
  [out_sel] -> Gateway Out6/1
  Delay1/1 -> [valid_out], data_valid/1
  [valid_out] -> Gateway Out2/1
  heap_pay_length/1 -> Assert4/1
  [spead_valid] -> Delay1/1
  Assert5/1 -> Concat5/2
  Assert4/1 -> [pld_len], Concat4/2
  Assert2/1 -> [heap_size], Concat3/2
  heap_size/1 -> Assert2/1
  time_stamp/1 -> Assert5/1
  Constant10/1 -> Concat5/1
  Constant2/1 -> Concat3/1
  Constant3/1 -> Concat/1
  Constant4/1 -> Concat/2
  Constant5/1 -> Concat/3
  Constant6/1 -> Concat/4
  Constant7/1 -> Concat/5
  Constant9/1 -> Concat4/1
  Concat/1 -> Mux/2
  Concat3/1 -> Mux/4
  Concat4/1 -> Mux/6
  Constant18/1 -> Concat9/1
  Assert10/1 -> Concat9/2

== system vegas13_fastnettest_250mhz_r1/sync_en ==
  sim_reg_in : Inport
  delay_pipe : Subsystem
  vegas13_fastnettest_250mhz_r1_sync_en_user_data_out : xbsIndex_r4/Gateway In  arith_type=Unsigned  n_bits=32  bin_pt=0  quantization="Round  (unbiased: +/- Inf)"  overflow=Saturate  period=1  dbl_ovrd=off  timing_constraint=None  locs_specified=off  LOCs={}  hdl_port=on  block_type=gatewayin
      settings: infoedit="Gateway in block.  Converts inputs of type Simulink integer, double and fixed point to  Xilinx fixed point type.<br><br>Hardware notes:  In hardware these blocks become top level input ports."  block_version=11.4
  reg_in : Outport
  wires:
  delay_pipe/1(q) -> reg_in/1
  vegas13_fastnettest_250mhz_r1_sync_en_user_data_out/1 -> delay_pipe/1(d)
  sim_reg_in/1 -> vegas13_fastnettest_250mhz_r1_sync_en_user_data_out/1

== system vegas13_fastnettest_250mhz_r1/sync_period ==
  sim_reg_in : Inport
  delay_pipe : Subsystem
  vegas13_fastnettest_250mhz_r1_sync_period_user_data_out : xbsIndex_r4/Gateway In  arith_type=Unsigned  n_bits=32  bin_pt=0  quantization="Round  (unbiased: +/- Inf)"  overflow=Saturate  period=1  dbl_ovrd=off  timing_constraint=None  locs_specified=off  LOCs={}  hdl_port=on  block_type=gatewayin
      settings: infoedit="Gateway in block.  Converts inputs of type Simulink integer, double and fixed point to  Xilinx fixed point type.<br><br>Hardware notes:  In hardware these blocks become top level input ports."  block_version=11.4
  reg_in : Outport
  wires:
  delay_pipe/1(q) -> reg_in/1
  vegas13_fastnettest_250mhz_r1_sync_period_user_data_out/1 -> delay_pipe/1(d)
  sim_reg_in/1 -> vegas13_fastnettest_250mhz_r1_sync_period_user_data_out/1

== system vegas13_fastnettest_250mhz_r1/sync_sel ==
  sim_reg_in : Inport
  delay_pipe : Subsystem
  vegas13_fastnettest_250mhz_r1_sync_sel_user_data_out : xbsIndex_r4/Gateway In  arith_type=Unsigned  n_bits=32  bin_pt=0  quantization="Round  (unbiased: +/- Inf)"  overflow=Saturate  period=1  dbl_ovrd=off  timing_constraint=None  locs_specified=off  LOCs={}  hdl_port=on  block_type=gatewayin
      settings: infoedit="Gateway in block.  Converts inputs of type Simulink integer, double and fixed point to  Xilinx fixed point type.<br><br>Hardware notes:  In hardware these blocks become top level input ports."  block_version=11.4
  reg_in : Outport
  wires:
  delay_pipe/1(q) -> reg_in/1
  vegas13_fastnettest_250mhz_r1_sync_sel_user_data_out/1 -> delay_pipe/1(d)
  sim_reg_in/1 -> vegas13_fastnettest_250mhz_r1_sync_sel_user_data_out/1

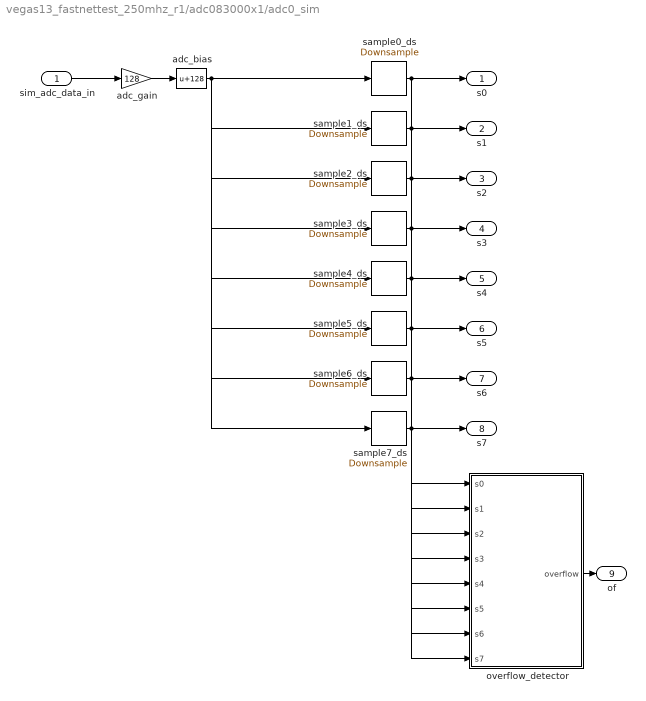
== system vegas13_fastnettest_250mhz_r1/adc083000x1/adc0_sim ==
  sim_adc_data_in : Inport  OutDataType=sfix(16)  OutScaling=2^0
  adc_bias : Bias  Bias=128  SaturateOnIntegerOverflow=on
  adc_gain : Gain  Gain=128  ParameterDataType=sfix(16)  ParameterScaling=2^0  OutDataType=sfix(16)  OutScaling=2^0
  overflow_detector : Subsystem  AncestorBlock=casper_library/Misc/of_detect_bus  mask(of_detect_bus){nStreams=8, bit_width=8}
      mask prompts: nStreams "Number of Streams"; bit_width "Bit Width"
      mask init:
      | adc_overflow_detector_init(gcb, ...
      |     'nStreams', nStreams, ...
      |     'bit_width', bit_width);
  sample0_ds : dspsigops/Downsample  N=8  phase=1  ic=0  smode=Force single rate  fmode=Maintain input frame size
  sample1_ds : dspsigops/Downsample  N=8  phase=2  ic=0  smode=Force single rate  fmode=Maintain input frame size
  sample2_ds : dspsigops/Downsample  N=8  phase=3  ic=0  smode=Force single rate  fmode=Maintain input frame size
  sample3_ds : dspsigops/Downsample  N=8  phase=4  ic=0  smode=Force single rate  fmode=Maintain input frame size
  sample4_ds : dspsigops/Downsample  N=8  phase=5  ic=0  smode=Force single rate  fmode=Maintain input frame size
  sample5_ds : dspsigops/Downsample  N=8  phase=6  ic=0  smode=Force single rate  fmode=Maintain input frame size
  sample6_ds : dspsigops/Downsample  N=8  phase=7  ic=0  smode=Force single rate  fmode=Maintain input frame size
  sample7_ds : dspsigops/Downsample  N=8  phase=0  ic=0  smode=Force single rate  fmode=Maintain input frame size
  s0 : Outport  OutDataType=sfix(16)  OutScaling=2^0
  s1 : Outport  Port=2  OutDataType=sfix(16)  OutScaling=2^0
  s2 : Outport  Port=3  OutDataType=sfix(16)  OutScaling=2^0
  s3 : Outport  Port=4  OutDataType=sfix(16)  OutScaling=2^0
  s4 : Outport  Port=5  OutDataType=sfix(16)  OutScaling=2^0
  s5 : Outport  Port=6  OutDataType=sfix(16)  OutScaling=2^0
  s6 : Outport  Port=7  OutDataType=sfix(16)  OutScaling=2^0
  s7 : Outport  Port=8  OutDataType=sfix(16)  OutScaling=2^0
  of : Outport  Port=9  OutDataType=sfix(16)  OutScaling=2^0
  wires:
  sim_adc_data_in/1 -> adc_gain/1
  adc_gain/1 -> adc_bias/1
  overflow_detector/1(overflow) -> of/1
  adc_bias/1 -> sample0_ds/1, sample1_ds/1, sample2_ds/1, sample3_ds/1, sample4_ds/1, sample5_ds/1, sample6_ds/1, sample7_ds/1
  sample0_ds/1 -> overflow_detector/1(s0), s0/1
  sample1_ds/1 -> overflow_detector/2(s1), s1/1
  sample2_ds/1 -> overflow_detector/3(s2), s2/1
  sample3_ds/1 -> overflow_detector/4(s3), s3/1
  sample4_ds/1 -> overflow_detector/5(s4), s4/1
  sample5_ds/1 -> overflow_detector/6(s5), s5/1
  sample6_ds/1 -> overflow_detector/7(s6), s6/1
  sample7_ds/1 -> overflow_detector/8(s7), s7/1

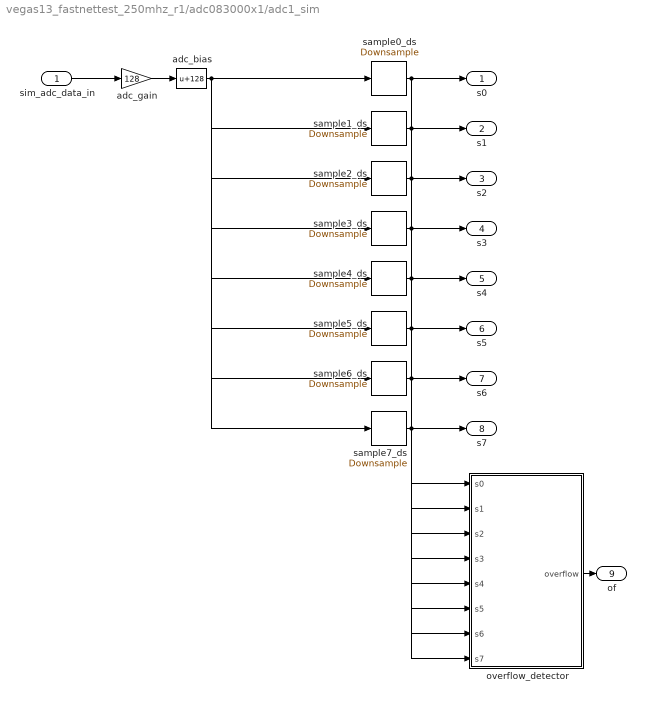
== system vegas13_fastnettest_250mhz_r1/adc083000x1/adc1_sim ==
  sim_adc_data_in : Inport  OutDataType=sfix(16)  OutScaling=2^0
  adc_bias : Bias  Bias=128  SaturateOnIntegerOverflow=on
  adc_gain : Gain  Gain=128  ParameterDataType=sfix(16)  ParameterScaling=2^0  OutDataType=sfix(16)  OutScaling=2^0
  overflow_detector : Subsystem  AncestorBlock=casper_library/Misc/of_detect_bus  mask(of_detect_bus){nStreams=8, bit_width=8}
      mask prompts: nStreams "Number of Streams"; bit_width "Bit Width"
      mask init:
      | adc_overflow_detector_init(gcb, ...
      |     'nStreams', nStreams, ...
      |     'bit_width', bit_width);
  sample0_ds : dspsigops/Downsample  N=8  phase=1  ic=0  smode=Force single rate  fmode=Maintain input frame size
  sample1_ds : dspsigops/Downsample  N=8  phase=2  ic=0  smode=Force single rate  fmode=Maintain input frame size
  sample2_ds : dspsigops/Downsample  N=8  phase=3  ic=0  smode=Force single rate  fmode=Maintain input frame size
  sample3_ds : dspsigops/Downsample  N=8  phase=4  ic=0  smode=Force single rate  fmode=Maintain input frame size
  sample4_ds : dspsigops/Downsample  N=8  phase=5  ic=0  smode=Force single rate  fmode=Maintain input frame size
  sample5_ds : dspsigops/Downsample  N=8  phase=6  ic=0  smode=Force single rate  fmode=Maintain input frame size
  sample6_ds : dspsigops/Downsample  N=8  phase=7  ic=0  smode=Force single rate  fmode=Maintain input frame size
  sample7_ds : dspsigops/Downsample  N=8  phase=0  ic=0  smode=Force single rate  fmode=Maintain input frame size
  s0 : Outport  OutDataType=sfix(16)  OutScaling=2^0
  s1 : Outport  Port=2  OutDataType=sfix(16)  OutScaling=2^0
  s2 : Outport  Port=3  OutDataType=sfix(16)  OutScaling=2^0
  s3 : Outport  Port=4  OutDataType=sfix(16)  OutScaling=2^0
  s4 : Outport  Port=5  OutDataType=sfix(16)  OutScaling=2^0
  s5 : Outport  Port=6  OutDataType=sfix(16)  OutScaling=2^0
  s6 : Outport  Port=7  OutDataType=sfix(16)  OutScaling=2^0
  s7 : Outport  Port=8  OutDataType=sfix(16)  OutScaling=2^0
  of : Outport  Port=9  OutDataType=sfix(16)  OutScaling=2^0
  wires:
  sim_adc_data_in/1 -> adc_gain/1
  adc_gain/1 -> adc_bias/1
  overflow_detector/1(overflow) -> of/1
  adc_bias/1 -> sample0_ds/1, sample1_ds/1, sample2_ds/1, sample3_ds/1, sample4_ds/1, sample5_ds/1, sample6_ds/1, sample7_ds/1
  sample0_ds/1 -> overflow_detector/1(s0), s0/1
  sample1_ds/1 -> overflow_detector/2(s1), s1/1
  sample2_ds/1 -> overflow_detector/3(s2), s2/1
  sample3_ds/1 -> overflow_detector/4(s3), s3/1
  sample4_ds/1 -> overflow_detector/5(s4), s4/1
  sample5_ds/1 -> overflow_detector/6(s5), s5/1
  sample6_ds/1 -> overflow_detector/7(s6), s6/1
  sample7_ds/1 -> overflow_detector/8(s7), s7/1

== system vegas13_fastnettest_250mhz_r1/arm/delay_pipe ==
  d : Inport
  q : Outport
  wires:
  d/1 -> q/1

== system vegas13_fastnettest_250mhz_r1/cnt_rst/delay_pipe ==
  d : Inport
  q : Outport
  wires:
  d/1 -> q/1

== system vegas13_fastnettest_250mhz_r1/dest_ip/delay_pipe ==
  d : Inport
  q : Outport
  wires:
  d/1 -> q/1

== system vegas13_fastnettest_250mhz_r1/dest_port/delay_pipe ==
  d : Inport
  q : Outport
  wires:
  d/1 -> q/1

== system vegas13_fastnettest_250mhz_r1/eth_rst/delay_pipe ==
  d : Inport
  q : Outport
  wires:
  d/1 -> q/1

== system vegas13_fastnettest_250mhz_r1/ip_select/delay_pipe ==
  d : Inport
  q : Outport
  wires:
  d/1 -> q/1

== system vegas13_fastnettest_250mhz_r1/port_select/delay_pipe ==
  d : Inport
  q : Outport
  wires:
  d/1 -> q/1
